simulink model "ArmModel1"  (R2017a)
settings: Solver=FixedStepAuto  StartTime=0.0  StopTime=84.77  FixedStep=0.01  RelTol=1e-3
undefined symbols (not defined in the file): DiscIntNeverNeededParam, sigbuilder_block
libraries: vrlib x8, sharedtransform x6, instrumentlib x1
settings Model: Creator=erich  LastModifiedBy=MarioAndres

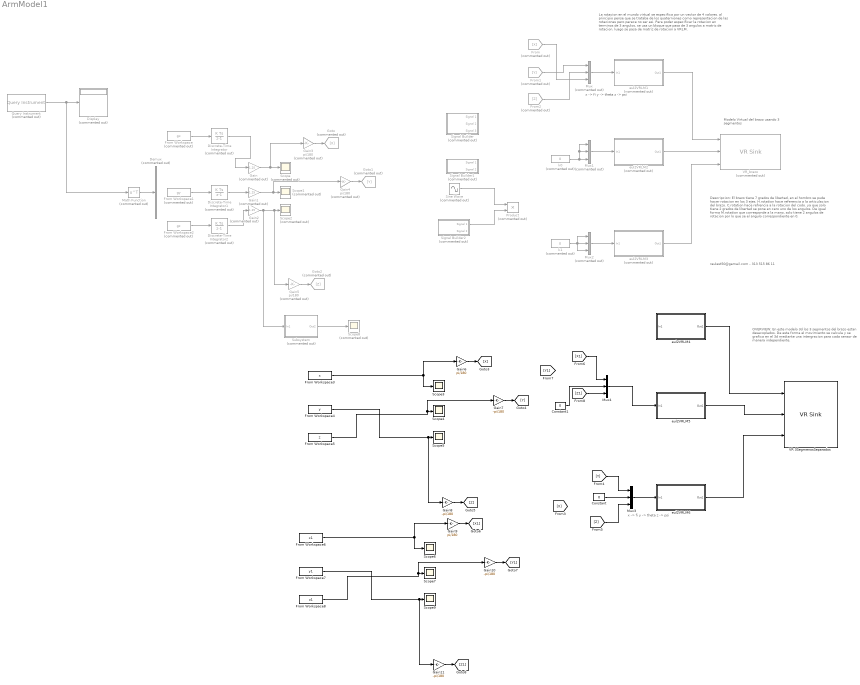
== system ArmModel1 ==
  note: La rotacion en el mundo virtual se especifica
      | por un vector de 4 valores. al principio pense que
      | se trataba de los quaterniones como representacion
      | de las rotaciones pero parece no ser asi. Para poder
      | especificar la rotacion en terminos de 3 angulos, se
      | usa un bloque que pasa de 3 angulos a matriz
      | de rotacion. luago se pasa de matriz de rotacion a
      | VRLM.
  note: Descripcion: El brazo tiene 7 grados
      | de libertad, en el hombro se pude
      | hacer rotacion en los 3 ejes.
      | H.rotation hace referencia a la articulacion del
      | brazo. C.rotation hace refrencia a la rotacion
      | del codo. ya que solo tiene 2 grados de libertad
      | se pone en cero uno de los angulos. De igual
      | forma M.rotation que corresponde a la mano,
      | solo tiene 2 angulos de rotacion por lo que se
      | el angulo correspondiente en 0.
  note: Modelo Virtual del brazo
      | usando 3 segmentos
  note: x -> fi
      | y -> theta
      | z -> psi
  note: raulest50@gamail.com - 313 515 86 11
  note: OVERVIEW:
      | En este modelo 3d los 3 segmentos del
      | brazo estan desacoplados. De esta forma
      | el movimiento se calcula y se grafica en el
      | 3d mediante una intergracion para cada
      | sensor de manera independiente.
  note: x -> fi
      | y -> theta
      | z -> psi
  Constant : Constant  Value=0
  Constant1 : Constant  Value=0
  Demux : Demux  Commented=on  Outputs=3
  Discrete-Time Integrator : DiscreteIntegrator  Commented=on  InitialConditionSetting=State (most efficient)  SampleTime=0.01  ICPrevOutput=DiscIntNeverNeededParam  ICPrevScaledInput=DiscIntNeverNeededParam
  Discrete-Time Integrator1 : DiscreteIntegrator  Commented=on  InitialConditionSetting=State (most efficient)  SampleTime=0.01  ICPrevOutput=DiscIntNeverNeededParam  ICPrevScaledInput=DiscIntNeverNeededParam
  Discrete-Time Integrator2 : DiscreteIntegrator  Commented=on  InitialConditionSetting=State (most efficient)  SampleTime=0.01  ICPrevOutput=DiscIntNeverNeededParam  ICPrevScaledInput=DiscIntNeverNeededParam
  Display : Display  Commented=on
  From : From  Commented=on  GotoTag=X
  From Workspace : FromWorkspace  Commented=on  VariableName=gx  SampleTime=0.01
  From Workspace1 : FromWorkspace  Commented=on  VariableName=gy  SampleTime=0.01
  From Workspace2 : FromWorkspace  Commented=on  VariableName=gz  SampleTime=0.01
  From Workspace3 : FromWorkspace  VariableName=x  SampleTime=0.01
  From Workspace4 : FromWorkspace  VariableName=y  SampleTime=0.01
  From Workspace5 : FromWorkspace  VariableName=z  SampleTime=0.01
  From Workspace6 : FromWorkspace  VariableName=x1  SampleTime=0.01
  From Workspace7 : FromWorkspace  VariableName=y1  SampleTime=0.01
  From Workspace8 : FromWorkspace  VariableName=z1  SampleTime=0.01
  From1 : From  Commented=on  GotoTag=Y
  From2 : From  Commented=on  GotoTag=Z
  Gain : Gain  Commented=on  Gain=1.25
  Gain1 : Gain  Commented=on  Gain=1.25
  Gain{7..8,10..11} (4 alike) : Gain  Gain=-pi/180
  Gain2 : Gain  Commented=on  Gain=1.25
  Gain3 : Gain  Commented=on  Gain=pi/180
  Gain4 : Gain  Commented=on  Gain=pi/180
  Gain5 : Gain  Commented=on  Gain=pi/180
  Gain6 : Gain  Gain=pi/180
  Gain9 : Gain  Gain=pi/180
  Goto : Goto  Commented=on  GotoTag=X
  Goto1 : Goto  Commented=on  GotoTag=Y
  Goto2 : Goto  Commented=on  GotoTag=Z
  Math Function : Math  Commented=on  Operator=transpose  OutputSignalType=real  SaturateOnIntegerOverflow=on
  Mux : Mux  Commented=on  Inputs=3
  Mux1 : Mux  Commented=on  Inputs=3
  Mux2 : Mux  Commented=on  Inputs=3
  Mux3 : Mux  Inputs=3
  Mux4 : Mux  Inputs=3
  Product : Product  Commented=on
  Query Instrument : instrumentlib/Query Instrument  Commented=on  sampleTime=0.01  isWorkspaceObject=off  timeout=10  inputBufferSize=512  protocol=Serial  serialPort=COM2  baudRate=115200  gpibVendor=Agilent Technologies  boardIndex=0  primaryAddress=1  secondaryAddress=0  visaVendor=Agilent  visaSerialPort=0  chassisIndex=0  logicalAddress=0  tcpRemoteHost='127.0.0.1'  tcpRemotePort=4500  udpRemoteHost='127.0.0.1'  udpRemotePort=9090  visaTCPBoardIndex=0  visaTCPRemoteHost='127.0.0.1'  usbBoardIndex=0  usbManufID=0  usbModelCode=0  usbSerialNumber=0  initAction=None  initCommand='DATA:SOURCE CH1'  initFunction=get  queryCommand='curve?'  responseFormat=ASCII  asciiFormatting='%f,'  precision=8-bit integer  byteOrder=Little endian  valuesToRead=1  removeBytes=off  afterOutputAction=Repeat query for new data  enableFrames=on  frameSize=3
      settings: SourceProductName=Instrument Control Toolbox  SourceProductBaseCode=IC
  Scope{,1..2,8} (4 alike) : Scope  Commented=on
  Scope{3..7,9} (6 alike) : Scope
  Signal Builder : Subsystem  Tag=STV Subsys  Commented=on  LoadFcn=sigbuilder_block('load');  StartFcn=sigbuilder_block('start');  StopFcn=sigbuilder_block('stop');  ClipboardFcn=sigbuilder_block('clipboard');  mask(Sigbuilder block){tuvar=[0:10]}
      mask help: Simulink:masks:SigbuilderBlock_MD
      mask init:
      | if ~strcmp(get_param(bdroot(gcbh),'SimulationStatus'),'stopped') tuvar = sigbuilder_block('maskInit'); end
      settings: CopyFcn=sigbuilder_block('copy');  DeleteFcn=sigbuilder_block('delete');  ModelCloseFcn=sigbuilder_block('modelClose');  PreSaveFcn=sigbuilder_block('preSave');  PauseFcn=sigbuilder_block('pause');  ContinueFcn=sigbuilder_block('continue');  NameChangeFcn=sigbuilder_block('namechange');  OpenFcn=sigbuilder_block('open',[437.25 153 550.5 359.25 ]);  CloseFcn=sigbuilder_block('close');
      mask Display: plot(0, 0, 100, 100,[2, 2, 32, 32, 2], [68, 8, 8, 68, 68],[32, 2], [38, 38], [32, 19, 2],[53, 60, 44], [32, 17, 17, 2],[16, 16, 31, 31]);txt = getActiveGroup(gcbh);text(2, 100, txt,'verticalAlignment', 'top');
  Signal Builder1 : Subsystem  Tag=STV Subsys  Commented=on  LoadFcn=sigbuilder_block('load');  StartFcn=sigbuilder_block('start');  StopFcn=sigbuilder_block('stop');  ClipboardFcn=sigbuilder_block('clipboard');  mask(Sigbuilder block){tuvar=[0:10]}
      mask help: Simulink:masks:SigbuilderBlock_MD
      mask init:
      | if ~strcmp(get_param(bdroot(gcbh),'SimulationStatus'),'stopped') tuvar = sigbuilder_block('maskInit'); end
      settings: CopyFcn=sigbuilder_block('copy');  DeleteFcn=sigbuilder_block('delete');  ModelCloseFcn=sigbuilder_block('modelClose');  PreSaveFcn=sigbuilder_block('preSave');  PauseFcn=sigbuilder_block('pause');  ContinueFcn=sigbuilder_block('continue');  NameChangeFcn=sigbuilder_block('namechange');  OpenFcn=sigbuilder_block('open',[437.25 153 550.5 359.25 ]);  CloseFcn=sigbuilder_block('close');
      mask Display: plot(0, 0, 100, 100,[2, 2, 32, 32, 2], [68, 8, 8, 68, 68],[32, 2], [38, 38], [32, 19, 2],[53, 60, 44], [32, 17, 17, 2],[16, 16, 31, 31]);txt = getActiveGroup(gcbh);text(2, 100, txt,'verticalAlignment', 'top');
  Signal Builder2 : Subsystem  Tag=STV Subsys  Commented=on  LoadFcn=sigbuilder_block('load');  StartFcn=sigbuilder_block('start');  StopFcn=sigbuilder_block('stop');  ClipboardFcn=sigbuilder_block('clipboard');  mask(Sigbuilder block){tuvar=[0:10]}
      mask help: Simulink:masks:SigbuilderBlock_MD
      mask init:
      | if ~strcmp(get_param(bdroot(gcbh),'SimulationStatus'),'stopped') tuvar = sigbuilder_block('maskInit'); end
      settings: CopyFcn=sigbuilder_block('copy');  DeleteFcn=sigbuilder_block('delete');  ModelCloseFcn=sigbuilder_block('modelClose');  PreSaveFcn=sigbuilder_block('preSave');  PauseFcn=sigbuilder_block('pause');  ContinueFcn=sigbuilder_block('continue');  NameChangeFcn=sigbuilder_block('namechange');  OpenFcn=sigbuilder_block('open',[437.25 153 550.5 359.25 ]);  CloseFcn=sigbuilder_block('close');
      mask Display: plot(0, 0, 100, 100,[2, 2, 32, 32, 2], [68, 8, 8, 68, 68],[32, 2], [38, 38], [32, 19, 2],[53, 60, 44], [32, 17, 17, 2],[16, 16, 31, 31]);txt = getActiveGroup(gcbh);text(2, 100, txt,'verticalAlignment', 'top');
  Sine Wave : Sin  Commented=on  Amplitude=pi/10  Frequency=3  SampleTime=0
  Subsystem : Subsystem  Commented=on
  VR 3SegmenosSeparados : vrlib/VR Sink  InstantiateOnLoad=on  SampleTime=0.01  ViewEnable=on  RemoteChange=off  RemoteView=off  FieldsWritten=Sphere_HombroCodo.rotation.4.1.1.double#Sphere_CodoMano.rotation.4.1.1.double#Sphere_Mano.rotation.4.1.1.double  WorldFileName=VM\VM_HCM_separados.wrl  AutoView=off  VideoDimensions=[]  AllowVariableSize=off
      settings: SourceProductBaseCode=VR
  VR_brazo : vrlib/VR Sink  Commented=on  InstantiateOnLoad=on  SampleTime=0.1  ViewEnable=on  RemoteChange=off  RemoteView=off  FieldsWritten=H.rotation.4.1.1.double#C.rotation.4.1.1.double#M.rotation.4.1.1.double  WorldFileName=Brazo_1.WRL  AutoView=off  VideoDimensions=[]  AllowVariableSize=off
      settings: SourceProductBaseCode=VR
  eul2VRLM1 : Subsystem  Commented=on
  eul2VRLM2 : Subsystem  Commented=on
  eul2VRLM3 : Subsystem  Commented=on
  eul2VRLM4 : Subsystem
  eul2VRLM5 : Subsystem
  eul2VRLM6 : Subsystem
  k0 : Constant  Commented=on  Value=0
  k1 : Constant  Commented=on  Value=0
  wires:
  Mux/1 -> eul2VRLM1/1(In1)
  eul2VRLM1/1(Out1) -> VR_brazo/1
  eul2VRLM2/1(Out1) -> VR_brazo/2
  eul2VRLM3/1(Out1) -> VR_brazo/3
  Mux1/1 -> eul2VRLM2/1(In1)
  Mux2/1 -> eul2VRLM3/1(In1)
  k0/1 -> Mux1/1, Mux1/2, Mux1/3
  k1/1 -> Mux2/1, Mux2/3, Mux2/2
  Sine Wave/1 -> Product/1
  Signal Builder2/1(Signal 1) -> Product/2
  Gain/1 -> Gain3/1, Scope/1
  Discrete-Time Integrator2/1 -> Gain2/1
  Discrete-Time Integrator/1 -> Gain/1
  Query Instrument/1 -> Display/1, Math Function/1
  Gain1/1 -> Gain4/1, Scope1/1
  Gain3/1 -> Goto/1
  Gain4/1 -> Goto1/1
  Gain5/1 -> Goto2/1
  From2/1 -> Mux/2
  From/1 -> Mux/3
  From1/1 -> Mux/1
  Discrete-Time Integrator1/1 -> Gain1/1
  Gain2/1 -> Subsystem/1(In1), Gain5/1, Scope2/1
  Subsystem/1(Out2) -> Scope8/1
  Math Function/1 -> Demux/1
  From Workspace/1 -> Discrete-Time Integrator/1
  From Workspace1/1 -> Discrete-Time Integrator1/1
  From Workspace2/1 -> Discrete-Time Integrator2/1
  From Workspace4/1 -> Scope5/1, Gain8/1
  Gain8/1 -> [Z]
  Gain7/1 -> [Y]
  Gain6/1 -> [X]
  From Workspace5/1 -> Scope4/1, Gain7/1
  From Workspace3/1 -> Scope3/1, Gain6/1
  eul2VRLM4/1(Out1) -> VR 3SegmenosSeparados/1
  eul2VRLM5/1(Out1) -> VR 3SegmenosSeparados/2
  eul2VRLM6/1(Out1) -> VR 3SegmenosSeparados/3
  From Workspace6/1 -> Gain9/1, Scope6/1
  From Workspace8/1 -> Gain10/1, Scope7/1
  Gain9/1 -> [X1]
  Gain10/1 -> [Y1]
  Gain11/1 -> [Z1]
  From Workspace7/1 -> Gain11/1, Scope9/1
  Mux3/1 -> eul2VRLM6/1(In1)
  Mux4/1 -> eul2VRLM5/1(In1)
  Constant/1 -> Mux3/2
  [Y] -> Mux3/1
  [Z] -> Mux3/3
  [X1] -> Mux4/1
  [Z1] -> Mux4/3
  Constant1/1 -> Mux4/2

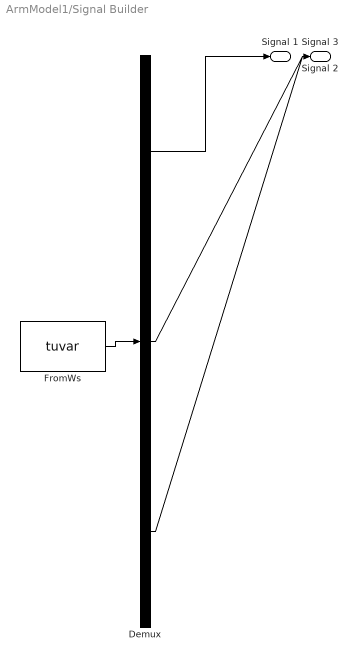
== system ArmModel1/Signal Builder ==
  Demux : Demux  Tag=STV Demux  Outputs=3
  FromWs : FromWorkspace  Tag=STV FromWs  VariableName=tuvar  SampleTime=0
      SigBuilderData=|
      | common.afterFinalStr = 'Extrapolate'
      | common.sampleTime = 0
      | dataSet.timeRange = [0 30]
      | dataSet.name = 'Group 1'
      | sbobj.Groups.Name = 'Group 1'
      | sbobj.Groups.Signals(1).Name = 'Signal 1'
      | sbobj.Groups.Signals(1).XData = [0 2 4 6 10 30]
      | sbobj.Groups.Signals(1).YData = [0 0 0.052 0.184 0.4 0.4]
      | sbobj.Groups.Signals(2).Name = 'Signal 2'
      | sbobj.Groups.Signals(2).XData = [0 30]
      | sbobj.Groups.Signals(2).YData = [0 0]
      | sbobj.Groups.Signals(3).Name = 'Signal 3'
      | sbobj.Groups.Signals(3).XData = [0 30]
      | sbobj.Groups.Signals(3).YData = [0 0]
      | sbobj.Groups.TimeRange = [0 30]
  Signal 1 : Outport  Tag=STV Outport
  Signal 2 : Outport  Tag=STV Outport  Port=2
  Signal 3 : Outport  Tag=STV Outport  Port=3
  wires:
  Demux/1 -> Signal 1/1
  FromWs/1 -> Demux/1
  Demux/2 -> Signal 2/1
  Demux/3 -> Signal 3/1

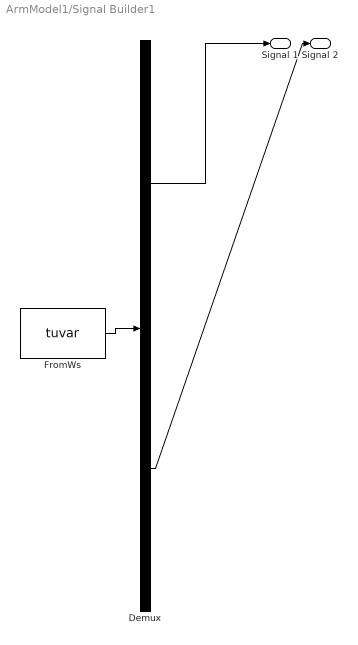
== system ArmModel1/Signal Builder1 ==
  Demux : Demux  Tag=STV Demux  Outputs=2
  FromWs : FromWorkspace  Tag=STV FromWs  VariableName=tuvar  SampleTime=0
      SigBuilderData=|
      | common.afterFinalStr = 'Extrapolate'
      | common.sampleTime = 0
      | dataSet.timeRange = [0 30]
      | dataSet.name = 'Group 1'
      | sbobj.Groups.Name = 'Group 1'
      | sbobj.Groups.Signals(1).Name = 'Signal 1'
      | sbobj.Groups.Signals(1).XData = [0 12 13 15 20 30]
      | sbobj.Groups.Signals(1).YData = [0 0 -0.255 -0.342 -0.308 -0.312]
      | sbobj.Groups.Signals(2).Name = 'Signal 2'
      | sbobj.Groups.Signals(2).XData = [0 30]
      | sbobj.Groups.Signals(2).YData = [0 0]
      | sbobj.Groups.TimeRange = [0 30]
  Signal 1 : Outport  Tag=STV Outport
  Signal 2 : Outport  Tag=STV Outport  Port=2
  wires:
  FromWs/1 -> Demux/1
  Demux/1 -> Signal 1/1
  Demux/2 -> Signal 2/1

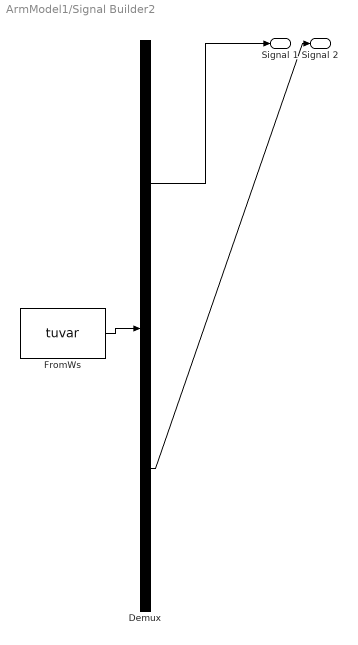
== system ArmModel1/Signal Builder2 ==
  Demux : Demux  Tag=STV Demux  Outputs=2
  FromWs : FromWorkspace  Tag=STV FromWs  VariableName=tuvar  SampleTime=0
      SigBuilderData=|
      | common.afterFinalStr = 'Extrapolate'
      | common.sampleTime = 0
      | dataSet.timeRange = [0 30]
      | dataSet.name = 'Group 1'
      | sbobj.Groups.Name = 'Group 1'
      | sbobj.Groups.Signals(1).Name = 'Signal 1'
      | sbobj.Groups.Signals(1).XData = [0 17 18 20 30]
      | sbobj.Groups.Signals(1).YData = [0 0 0.91 1 1]
      | sbobj.Groups.Signals(2).Name = 'Signal 2'
      | sbobj.Groups.Signals(2).XData = [0 30]
      | sbobj.Groups.Signals(2).YData = [0 0]
      | sbobj.Groups.TimeRange = [0 30]
  Signal 1 : Outport  Tag=STV Outport
  Signal 2 : Outport  Tag=STV Outport  Port=2
  wires:
  Demux/1 -> Signal 1/1
  FromWs/1 -> Demux/1
  Demux/2 -> Signal 2/1

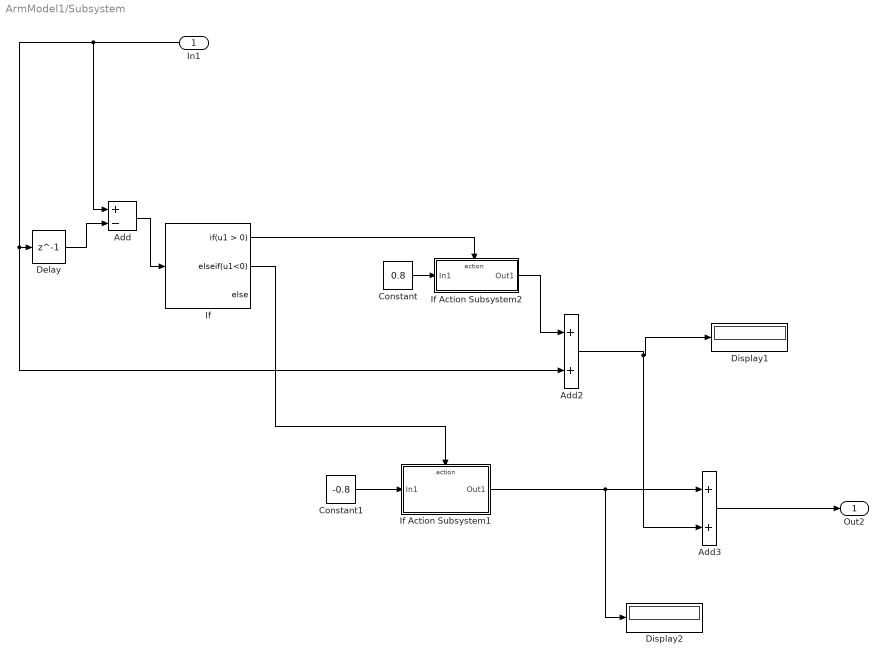
== system ArmModel1/Subsystem ==
  In1 : Inport
  Add : Sum  Inputs=+-
  Add2 : Sum
  Add3 : Sum
  Constant : Constant  Value=0.8
  Constant1 : Constant  Value=-0.8
  Delay : Delay  DelayLength=1  InitialCondition=0  SampleTime=0.01
  Display1 : Display
  Display2 : Display
  If : If  ElseIfExpressions=u1<0
  If Action Subsystem1 : Subsystem  TreatAsAtomicUnit=on
  If Action Subsystem2 : Subsystem  TreatAsAtomicUnit=on
  Out2 : Outport
  wires:
  Delay/1 -> Add/2
  If/1 -> If Action Subsystem2/Action
  Add/1 -> If/1
  If/2 -> If Action Subsystem1/Action
  If Action Subsystem1/1(Out1) -> Display2/1, Add3/1
  Add2/1 -> Display1/1, Add3/2
  Constant1/1 -> If Action Subsystem1/1(In1)
  Add3/1 -> Out2/1
  Constant/1 -> If Action Subsystem2/1(In1)
  If Action Subsystem2/1(Out1) -> Add2/1
  In1/1 -> Add/1, Add2/2, Delay/1

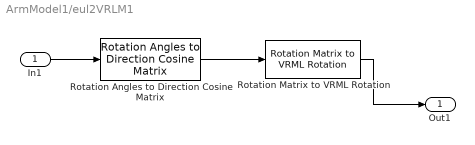
== system ArmModel1/eul2VRLM1 ==
  In1 : Inport
  Rotation Angles to Direction Cosine Matrix : sharedtransform/Rotation Angles to Direction Cosine Matrix  rotationOrder=ZYX
  Rotation Matrix to VRML Rotation : vrlib/Utilities/Rotation Matrix to VRML Rotation  maxzero=1e-12
      settings: SourceProductName=Simulink 3D Animation  SourceProductBaseCode=VR
  Out1 : Outport
  wires:
  Rotation Matrix to VRML Rotation/1 -> Out1/1
  In1/1 -> Rotation Angles to Direction Cosine Matrix/1
  Rotation Angles to Direction Cosine Matrix/1 -> Rotation Matrix to VRML Rotation/1

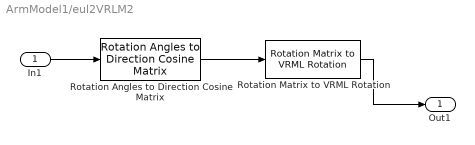
== system ArmModel1/eul2VRLM2 ==
  In1 : Inport
  Rotation Angles to Direction Cosine Matrix : sharedtransform/Rotation Angles to Direction Cosine Matrix  rotationOrder=ZYX
  Rotation Matrix to VRML Rotation : vrlib/Utilities/Rotation Matrix to VRML Rotation  maxzero=1e-12
      settings: SourceProductName=Simulink 3D Animation  SourceProductBaseCode=VR
  Out1 : Outport
  wires:
  Rotation Angles to Direction Cosine Matrix/1 -> Rotation Matrix to VRML Rotation/1
  In1/1 -> Rotation Angles to Direction Cosine Matrix/1
  Rotation Matrix to VRML Rotation/1 -> Out1/1

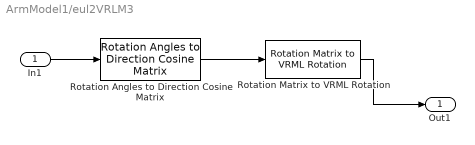
== system ArmModel1/eul2VRLM3 ==
  In1 : Inport
  Rotation Angles to Direction Cosine Matrix : sharedtransform/Rotation Angles to Direction Cosine Matrix  rotationOrder=ZYX
  Rotation Matrix to VRML Rotation : vrlib/Utilities/Rotation Matrix to VRML Rotation  maxzero=1e-12
      settings: SourceProductName=Simulink 3D Animation  SourceProductBaseCode=VR
  Out1 : Outport
  wires:
  Rotation Matrix to VRML Rotation/1 -> Out1/1
  In1/1 -> Rotation Angles to Direction Cosine Matrix/1
  Rotation Angles to Direction Cosine Matrix/1 -> Rotation Matrix to VRML Rotation/1

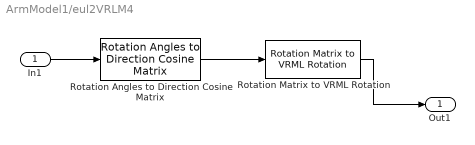
== system ArmModel1/eul2VRLM4 ==
  In1 : Inport
  Rotation Angles to Direction Cosine Matrix : sharedtransform/Rotation Angles to Direction Cosine Matrix  rotationOrder=ZYX
  Rotation Matrix to VRML Rotation : vrlib/Utilities/Rotation Matrix to VRML Rotation  maxzero=1e-12
      settings: SourceProductName=Simulink 3D Animation  SourceProductBaseCode=VR
  Out1 : Outport
  wires:
  Rotation Matrix to VRML Rotation/1 -> Out1/1
  In1/1 -> Rotation Angles to Direction Cosine Matrix/1
  Rotation Angles to Direction Cosine Matrix/1 -> Rotation Matrix to VRML Rotation/1

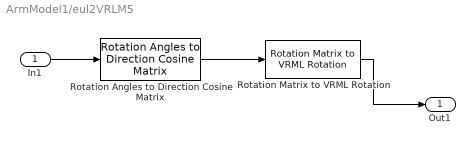
== system ArmModel1/eul2VRLM5 ==
  In1 : Inport
  Rotation Angles to Direction Cosine Matrix : sharedtransform/Rotation Angles to Direction Cosine Matrix  rotationOrder=ZYX
  Rotation Matrix to VRML Rotation : vrlib/Utilities/Rotation Matrix to VRML Rotation  maxzero=1e-12
      settings: SourceProductName=Simulink 3D Animation  SourceProductBaseCode=VR
  Out1 : Outport
  wires:
  Rotation Angles to Direction Cosine Matrix/1 -> Rotation Matrix to VRML Rotation/1
  In1/1 -> Rotation Angles to Direction Cosine Matrix/1
  Rotation Matrix to VRML Rotation/1 -> Out1/1

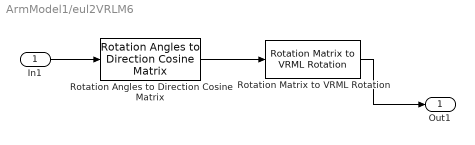
== system ArmModel1/eul2VRLM6 ==
  In1 : Inport
  Rotation Angles to Direction Cosine Matrix : sharedtransform/Rotation Angles to Direction Cosine Matrix  rotationOrder=ZYX
  Rotation Matrix to VRML Rotation : vrlib/Utilities/Rotation Matrix to VRML Rotation  maxzero=1e-12
      settings: SourceProductName=Simulink 3D Animation  SourceProductBaseCode=VR
  Out1 : Outport
  wires:
  Rotation Matrix to VRML Rotation/1 -> Out1/1
  In1/1 -> Rotation Angles to Direction Cosine Matrix/1
  Rotation Angles to Direction Cosine Matrix/1 -> Rotation Matrix to VRML Rotation/1

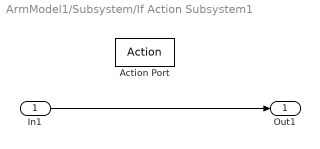
== system ArmModel1/Subsystem/If Action Subsystem1 ==
  In1 : Inport
  Action Port : ActionPort  ActionType=elseif
  Out1 : Outport
  wires:
  In1/1 -> Out1/1

== system ArmModel1/Subsystem/If Action Subsystem2 ==
  In1 : Inport
  Action Port : ActionPort  ActionType=then
  Out1 : Outport
  wires:
  In1/1 -> Out1/1
